simulink model "kalman_filter"  (R2024b)
settings: Solver=ode45  StartTime=0.0  StopTime=10  RelTol=1e-3
settings Model: Creator=apple  LastModifiedBy=apple

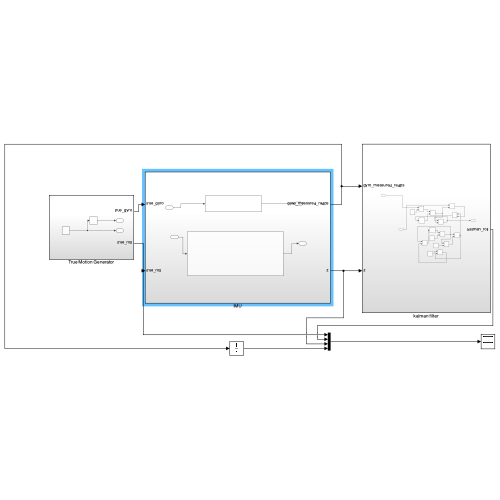
[thumbnail: Simulink's stored preview of the top-level diagram]
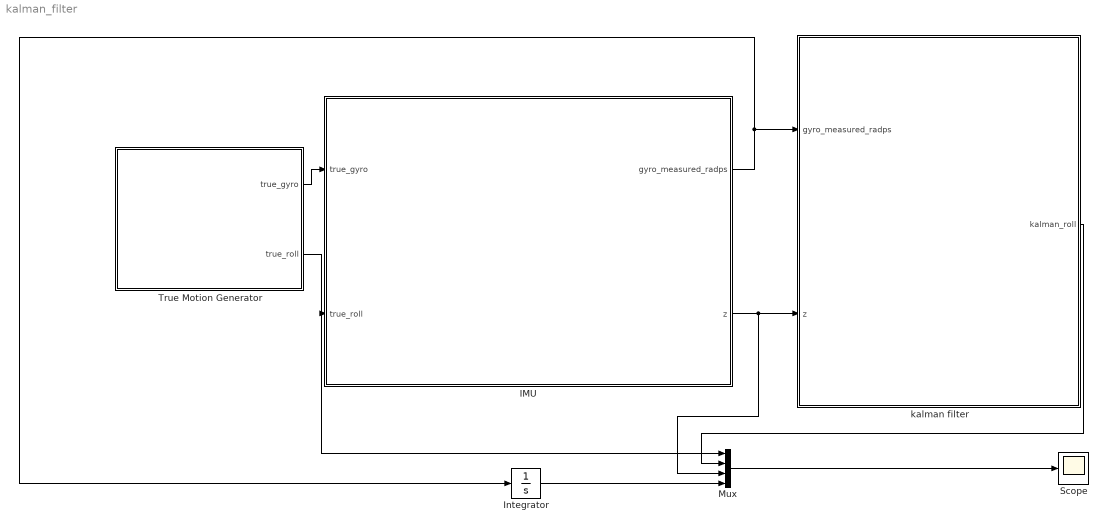
== system kalman_filter ==
  IMU : Subsystem
  Integrator : Integrator
  Mux : Mux
  Scope : Scope
  True Motion Generator : Subsystem
  kalman filter : Subsystem
  wires:
  Mux/1 -> Scope/1
  True Motion Generator/2(true_roll) -> IMU/2(true_roll), Mux/1
  kalman filter/1(kalman_roll) -> Mux/2
  Integrator/1 -> Mux/4
  IMU/2(z) -> Mux/3, kalman filter/2(z)
  IMU/1(gyro_measured_radps) -> kalman filter/1(gyro_measured_radps), Integrator/1
  True Motion Generator/1(true_gyro) -> IMU/1(true_gyro)

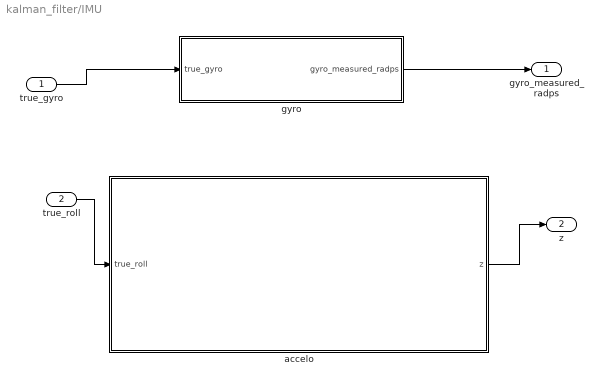
== system kalman_filter/IMU ==
  true_gyro : Inport
  true_roll : Inport  Port=2
  accelo : Subsystem
  gyro : Subsystem
  gyro_measured_radps : Outport
  z : Outport  Port=2
  wires:
  gyro/1(gyro_measured_radps) -> gyro_measured_radps/1
  accelo/1(z) -> z/1
  true_gyro/1 -> gyro/1(true_gyro)
  true_roll/1 -> accelo/1(true_roll)

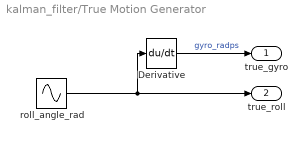
== system kalman_filter/True Motion Generator ==
  Derivative : Derivative
  roll_angle_rad : Sin  Amplitude=pi/4  SampleTime=0
  true_gyro : Outport
  true_roll : Outport  Port=2
  wires:
  Derivative/1 -> true_gyro/1  "gyro_radps"
  roll_angle_rad/1 -> true_roll/1, Derivative/1

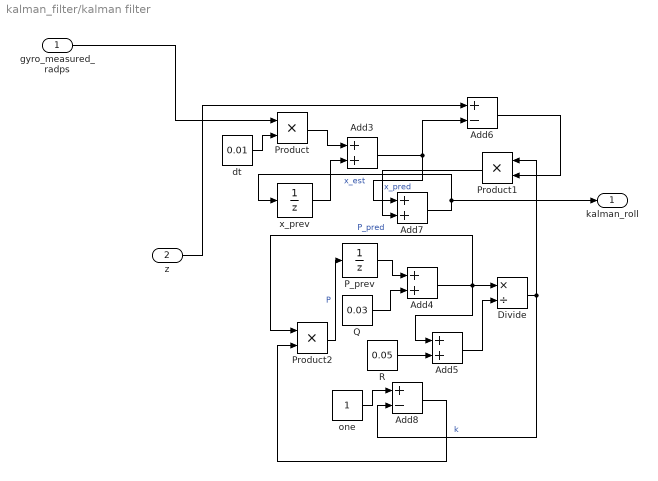
== system kalman_filter/kalman filter ==
  gyro_measured_radps : Inport
  z : Inport  Port=2
  Add{3..5,7} (4 alike) : Sum
  Add6 : Sum  Inputs=+-
  Add8 : Sum  Inputs=+-
  Divide : Product  Inputs=*/
  P_prev : UnitDelay  SampleTime=-1  HasFrameUpgradeWarning=on
  Product : Product
  Product1 : Product
  Product2 : Product
  Q : Constant  Value=0.03
  R : Constant  Value=0.05
  dt : Constant  Value=0.01
  one : Constant
  x_prev : UnitDelay  SampleTime=-1  HasFrameUpgradeWarning=on
  kalman_roll : Outport
  wires:
  gyro_measured_radps/1 -> Product/1
  Add5/1 -> Divide/2
  z/1 -> Add6/1
  Divide/1 -> Product1/1, Add8/2  "k"
  P_prev/1 -> Add4/1
  Product1/1 -> Add7/2
  R/1 -> Add5/2
  Product/1 -> Add3/1
  dt/1 -> Product/2
  Product2/1 -> P_prev/1  "P"
  x_prev/1 -> Add3/2
  Add6/1 -> Product1/2
  Q/1 -> Add4/2
  Add4/1 -> Product2/1, Divide/1, Add5/1  "P_pred"
  Add8/1 -> Product2/2
  one/1 -> Add8/1
  Add7/1 -> kalman_roll/1, x_prev/1  "x_est"
  Add3/1 -> Add6/2, Add7/1  "x_pred"

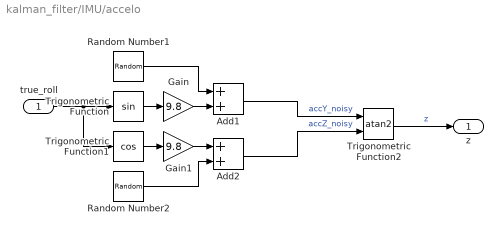
== system kalman_filter/IMU/accelo ==
  true_roll : Inport
  Add1 : Sum
  Add2 : Sum
  Gain : Gain  Gain=9.8
  Gain1 : Gain  Gain=9.8
  Random Number1 : RandomNumber  Variance=0.01  SampleTime=0.1
  Random Number2 : RandomNumber  Variance=0.01  SampleTime=0.1
  Trigonometric Function : Trigonometry
  Trigonometric Function1 : Trigonometry  Operator=cos
  Trigonometric Function2 : Trigonometry  Operator=atan2
  z : Outport
  wires:
  true_roll/1 -> Trigonometric Function1/1, Trigonometric Function/1
  Add2/1 -> Trigonometric Function2/2  "accZ_noisy"
  Trigonometric Function1/1 -> Gain1/1
  Gain/1 -> Add1/2
  Trigonometric Function2/1 -> z/1  "z"
  Random Number1/1 -> Add1/1
  Gain1/1 -> Add2/1
  Add1/1 -> Trigonometric Function2/1  "accY_noisy"
  Trigonometric Function/1 -> Gain/1
  Random Number2/1 -> Add2/2

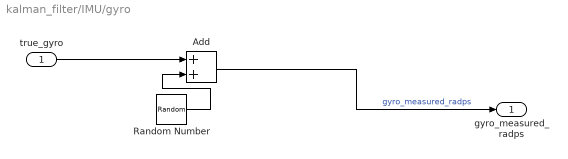
== system kalman_filter/IMU/gyro ==
  true_gyro : Inport
  Add : Sum
  Random Number : RandomNumber  Variance=0.01  SampleTime=0.1
  gyro_measured_radps : Outport
  wires:
  true_gyro/1 -> Add/1
  Add/1 -> gyro_measured_radps/1  "gyro_measured_radps"
  Random Number/1 -> Add/2
